simulink model "main_model_fd_v05_energyprotect"  (R2025a)
settings: Solver=ode3  StartTime=0.0  StopTime=1.5  FixedStep=1e-6  RelTol=1e-3
model workspace (MAT data in the model file):
  EP_ENERGY_INITIAL = 176
  EP_PBAT_SIGN = 1
  EP_PLOAD_SIGN = -1
  EP_POWER_ALPHA = 0.951229424501
  EP_POWER_BALANCE_ALPHA = 0.951229424501
  EP_POWER_CONFIRM_TIME = 0.01
  EP_POWER_FILTER_TAU = 0.002
  EP_PSOURCE_SIGN = 1
  EP_P_CHARGE_TRIP = 3000
  EP_P_CHARGE_WARN = 2500
  EP_P_DISCHARGE_TRIP = 3000
  EP_P_DISCHARGE_WARN = 2500
  EP_SOC_CHARGE_RELEASE = 88
  EP_SOC_CHARGE_STOP = 90
  EP_SOC_DISCHARGE_RELEASE = 12
  EP_SOC_DISCHARGE_STOP = 10
  EP_SOC_WARN_HIGH = 85
  EP_SOC_WARN_LOW = 15
  EP_TS = 0.0001
  FD_CBUS = 0.0022
  FD_CBUS_ESR = 0.001
  FD_CURRENT_QUANT_STEP = 1e-06
  FD_DUTY_BIAS = 0
  FD_DUTY_STUCK_ENABLE = 0
  FD_DUTY_STUCK_VALUE = 0.5
  FD_FAULT_END_TIME = 1000000000
  FD_FAULT_ID = 0
  FD_FAULT_TIME = 0.8
  FD_IBAT_BIAS = 0
  FD_IBAT_NOISE_STD = 0
  FD_IBAT_TRIP = 20
  FD_IL_BIAS = 0
  FD_IL_NOISE_STD = 0
  FD_IL_TRIP = 15
  FD_IREF_LEVEL = 10
  FD_IREF_OVERRIDE_ENABLE = 0
  FD_LOAD_STEP_A = 0
  FD_LOAD_STEP_TIME = 0.5
  FD_L_MAIN = 0.015
  FD_MODE_COMMAND = 2
  FD_MODE_OVERRIDE_ENABLE = 0
  FD_PROTECTION_ARM_TIME = 0.15
  FD_PROTECTION_MODE = 2
  FD_RBAT = 0.5
  FD_S1_FAULT_PULSE_WIDTH = 0
  FD_S1_OPEN = 0
  FD_S2_FAULT_PULSE_WIDTH = 0
  FD_S2_OPEN = 0
  FD_SENSOR_TS = 5e-05
  FD_SWITCH_FAULT_PERIOD = 0.0005
  FD_TRIP_DELAY_STEPS = 20000
  FD_TS = 1e-06
  FD_VBAT_BIAS = 0
  FD_VBAT_NOISE_STD = 0
  FD_VBAT_QUANT_STEP = 1e-06
  FD_VBUS_BIAS = 0
  FD_VBUS_HI = 430
  FD_VBUS_LO = 360
  FD_VBUS_NOISE_STD = 0
  FD_VBUS_QUANT_STEP = 1e-06
  I_charge_max = 10
  I_discharge_cmd = 10
  RandomSeed = 240727
  SOCInit = 20
  Var10 = 0
  Var11 = 0
  Var6 = 0
  Var7 = 0
  Var8 = 0
  Var9 = 0
undefined symbols (not defined in the file): DiscIntNeverNeededParam, dspblkCoreblockFVToolHelper, gcbh, Ion, Lithium
libraries: hdlsllib x17, spsSeriesRLCBranchLib x6, spsCurrentMeasurementLib x3, simulink x2, spsIGBTDiodeLib x2, eeGeneralControl x2, slpidlib x2, spsVoltageMeasurementLib x2, spsBatteryLib x1, spsControlledVoltageSourceLib x1, spsControlledCurrentSourceLib x1, spsPWMGeneratorDCDCLib x1
(part 1 of 2)
settings Model: Creator=Limingyu  LastModifiedBy=Administrator
settings DataIOCC: SaveState=on

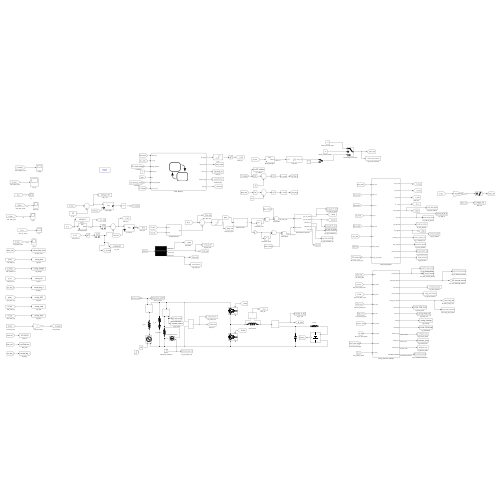
[thumbnail: Simulink's stored preview of the top-level diagram]
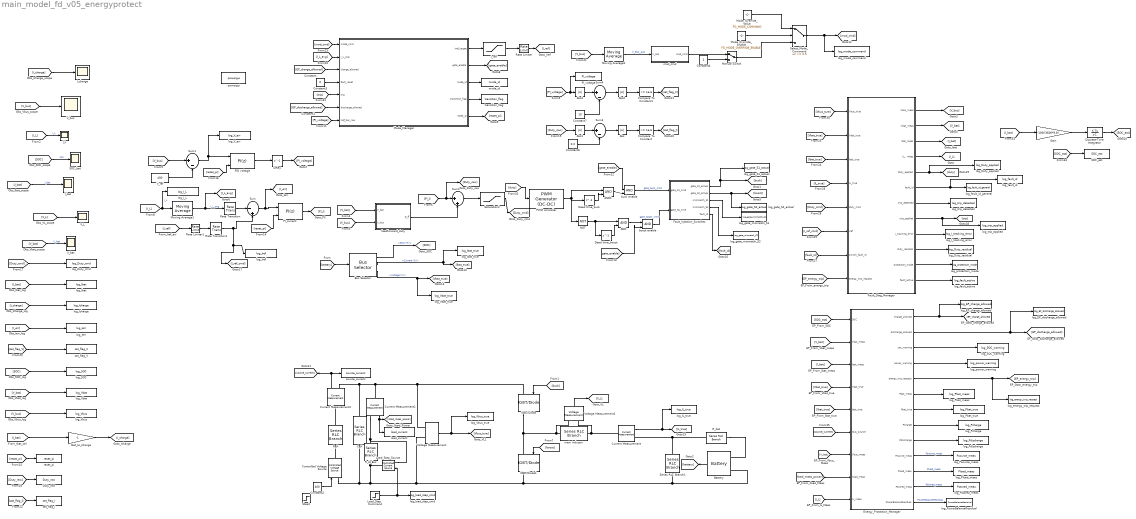
== system main_model_fd_v05_energyprotect ==
  AND : Logic  IconShape=distinctive  AllPortsSameDT=off  OutDataTypeStr=boolean
  AND1 : Logic  IconShape=distinctive  AllPortsSameDT=off  OutDataTypeStr=boolean
  Abs{,1..3} (4 alike) : Abs  SaturateOnIntegerOverflow=off
  Battery : spsBatteryLib/Battery  BatType=Lithium-Ion  NomV=200  NomQ=9.8  SOC=20  Batt_Tr=30  PresetModel=on  MaxQ=9.8  MinV=150  FullV=232.7974  Dis_rate=4.2609  R=0.20408  Normal_OP=8.8626  expZone="[216.0772     0.4814783]"
      link override Model/Discrete/Unit Delay: InitialCondition=Batt.E0 - Batt.K*Batt.Q/(Batt.Q-(1-SOC/100)*Batt.Q*(1/Batt.lambda))*((1-SOC/100)*Batt.Q*(1/Batt.lambda)) + Batt.A*exp(-Batt.B*((1-SOC/100)*Batt.Q*(1/Batt.lambda)))
  Bus Selector : BusSelector  OutputSignals=SOC (%),Current (A),Voltage (V)
  C_H : spsSeriesRLCBranchLib/Series RLC Branch  LConnTagsString=__new0  RConnTagsString=__new0  BranchType=RC  Resistance=FD_CBUS_ESR  Inductance=1e-3  SetiL0=off  InitialCurrent=0  Capacitance=FD_CBUS  Setx0=on  InitialVoltage=400  Measurements=Branch voltage
  Compare To Constant : simulink/Logic and Bit Operations/Compare To Constant  relop=<=  const=1e-6  OutDataTypeStr=boolean
  Compare To Constant1 : simulink/Logic and Bit Operations/Compare To Constant  relop=<=  const=1e-6  OutDataTypeStr=boolean
  Constant2 : Constant  Value=400
  Constant3 : Constant  Value=0  OutDataTypeStr=boolean
  Constant4 : Constant  OutDataTypeStr=double
  Constant6 : Constant  Value=0.2
  Constant7 : Constant  Value=10
  Controlled Voltage Source : spsControlledVoltageSourceLib/Controlled Voltage Source  Initialize=on  Source_Type=DC  Amplitude=400  Phase=0  Frequency=0  Measurements=None
  Current Measurement : spsCurrentMeasurementLib/Current Measurement  PhasorSimulation=off  OutputType=Complex  PSBequivalent=0
  Current Measurement1 : spsCurrentMeasurementLib/Current Measurement  PhasorSimulation=off  OutputType=Complex  PSBequivalent=0
  Current Measurement2 : spsCurrentMeasurementLib/Current Measurement  PhasorSimulation=off  OutputType=Complex  PSBequivalent=0
  Dead time_boost : Delay  DelayLength=1  InputProcessing=Columns as channels (frame based)  SampleTime=2e-6
  Dead time_buck : Delay  DelayLength=1  InputProcessing=Columns as channels (frame based)  SampleTime=2e-6
  Delay : Delay  DelayLength=1  InputProcessing=Columns as channels (frame based)  SampleTime=1e-3
  Discrete-Time Integrator : DiscreteIntegrator  InitialCondition=SOCInit  SampleTime=EP_TS  LimitOutput=on  UpperSaturationLimit=100  LowerSaturationLimit=0  ICPrevOutput=DiscIntNeverNeededParam  ICPrevScaledInput=DiscIntNeverNeededParam
  Duty_raw : ToWorkspace  VariableName=Duty_raw  SaveFormat=Timeseries  SampleTime=-1
  Energy_Protection_Manager : Subsystem
  Fault_Diag_Manager : Subsystem
  Fault_Injection_Switches : Subsystem
  Gain : Gain  Gain=-100/(3600*9.8)
  IGBT/Diode : spsIGBTDiodeLib/IGBT//Diode  Ron=1e-3  Rs=1e5  Cs=inf  Measurements=on
  IGBT/Diode1 : spsIGBTDiodeLib/IGBT//Diode  Ron=1e-3  Rs=1e5  Cs=inf  Measurements=on
  I_L : Scope
      settings: ActiveDisplayYMinimum=-1  ActiveDisplayYMaximum=1
  I_bat : Scope
      settings: ActiveDisplayYMinimum=9.9262651650151241  ActiveDisplayYMaximum=26.223015826126126  DataLoggingVariableName=scope_V_bat1
  I_charge : Scope
      settings: ActiveDisplayYMinimum=-1435.850063928573  ActiveDisplayYMaximum=6954.7870735806873  DataLoggingVariableName=scope_I_L
  I_ref' : Saturate  UpperLimit=I_charge_max  LowerLimit=-I_discharge_cmd
  Ibat_to_Icharge : Gain  Gain=-1
  Load_Step_Command : Step  Time=FD_LOAD_STEP_TIME  After=FD_LOAD_STEP_A  SampleTime=FD_TS
  Load_Step_Source : spsControlledCurrentSourceLib/Controlled Current Source  Initialize=on  Source_Type=AC  Amplitude=0  Phase=0  Frequency=0  Measurements=None
  Manual Switch : ManualSwitch
  Mode_Manager : Stateflow chart  TreatAsAtomicUnit=on
  Mode_Override_Enable : Constant  Value=FD_MODE_OVERRIDE_ENABLE
  Mode_Override_Value : Constant  Value=FD_MODE_COMMAND
  Moving Average1 : eeGeneralControl/Moving Average  VariantControl=Variant1  LabelModeActiveChoice=Discrete  f=20e3  x0=0  BufferSize=8192  Ts=1e-6
      settings: LibrarySourceBlock=ee_sl_lib/General Control/Moving Average
  Moving Average2 : eeGeneralControl/Moving Average  VariantControl=Variant1  LabelModeActiveChoice=Discrete  f=20e3  x0=0  BufferSize=8192  Ts=1e-6
      settings: LibrarySourceBlock=ee_sl_lib/General Control/Moving Average
  NOT : Logic  Operator=NOT  IconShape=distinctive  AllPortsSameDT=off  OutDataTypeStr=boolean
  PID voltage : slpidlib/PID Controller  Controller=PI  Form=Parallel  TimeDomain=Discrete-time  UseExternalTs=off  SampleTime=1e-3  IntegratorMethod=Forward Euler  FilterMethod=Forward Euler  ControllerParametersSource=internal  P=2.6  I=50  UseKiTs=off  D=0  UseExternalDerivativeSource=off  N=100  UseFilter=on  TunerSelectOption=Transfer Function Based (PID Tuner App)  InitialConditionSource=internal  InitialConditionForIntegrator=0  InitialConditionForFilter=0  DifferentiatorICPrevScaledInput=0  ExternalReset=rising  TrackingMode=off  Kt=1  LimitOutput=on  SatLimitsSource=internal  UpperSaturationLimit=10  LowerSaturationLimit=-10  LinearizeAsGain=on  AntiWindupMode=back-calculation  Kb=20  LimitIntegrator=off  UpperIntegratorSaturationLimit=inf  LowerIntegratorSaturationLimit=-inf  POutMin=[]  POutMax=[]  IOutMin=[]  IOutMax=[]  DOutMin=[]  DOutMax=[]  NOutMin=[]  NOutMax=[]  SumOutMin=[]  SumOutMax=[]  SaturationOutMin=[]  SaturationOutMax=[]  PParamMin=[]  PParamMax=[]  IParamMin=[]  IParamMax=[]  DParamMin=[]  DParamMax=[]  NParamMin=[]  NParamMax=[]  KbParamMin=[]  KbParamMax=[]  KtParamMin=[]  KtParamMax=[]  KbOutMin=[]  KbOutMax=[]  KtOutMin=[]  KtOutMax=[]  IntegratorOutMin=[]  IntegratorOutMax=[]  FilterOutMin=[]  FilterOutMax=[]  SumI1OutMin=[]  SumI1OutMax=[]  SumI2OutMin=[]  SumI2OutMax=[]  SumI3OutMin=[]  SumI3OutMax=[]  SumI4OutMin=[]  SumI4OutMax=[]  SumDOutMin=[]  SumDOutMax=[]  DifferentiatorOutMin=[]  DifferentiatorOutMax=[]  FilterDiffOutCoefMin=[]  FilterDiffOutCoefMax=[]  ReciprocalOutMin=[]  ReciprocalOutMax=[]  SumDenOutMin=[]  SumDenOutMax=[]  SumNumOutMin=[]  SumNumOutMax=[]  DivideOutMin=[]  DivideOutMax=[]  UdiffTsProdOutMin=[]  UdiffTsProdOutMax=[]  NTsProdOutMin=[]  NTsProdOutMax=[]  UintegralTsProdOutMin=[]  UintegralTsProdOutMax=[]  UngainTsProdOutMin=[]  UngainTsProdOutMax=[]  ClampingZeroOutDataTypeStr=Inherit: Inherit via back propagation  ClampingZeroOutMin=[]  ClampingZeroOutMax=[]  FilterDenConstantOutDataTypeStr=Inherit: Inherit via back propagation  FilterDenConstantOutMin=[]  FilterDenConstantOutMax=[]  PCopyOutDataTypeStr=Inherit: Inherit via back propagation  PCopyOutMin=[]  PCopyOutMax=[]  NCopyOutDataTypeStr=Inherit: Inherit via back propagation  NCopyOutMin=[]  NCopyOutMax=[]  IntegratorContinuousStateAttributes=''  IntegratorStateMustResolveToSignalObject=off  IntegratorRTWStateStorageClass=Auto  FilterContinuousStateAttributes=''  FilterStateMustResolveToSignalObject=off  FilterRTWStateStorageClass=Auto  ParallelPVariant=InternalParameters  IdealPVariant=Disabled  IVariant=InternalParameters  DVariant=Disabled  IntegratorVariant=Discrete  SatVariant=Enabled  AWVariant=BackCalculation  PCopyVariant=Disabled  TRVariant=Disabled  FdbkBlocksVariant=Forward  IdealPFdbkVariant=Disabled  SatFdbkVariant=Disabled  DerivativeFilterVariant=Disabled  NVariant=Disabled  NCopyVariant=Disabled_SignalSpec  FilterICVariant=Disabled  IntegratorICVariant=InternalICs  ExternalResetVariant=ExternalReset  TRSumVariant=Passthrough  SumFdbkVariant=Disabled  SumVariant=Sum_PI  TsampFilterVariant=InternalTs  TsampNgainVariant=Passthrough  TsampIntegralVariant=Disabled_SignalSpec  ExternalSaturationOutDataTypeStr=Inherit: Same as second input  DerivativeSourceVariant=Disabled  PreIntVariant=InternalPreInt
  PI_current : slpidlib/PID Controller  Controller=PI  Form=Parallel  TimeDomain=Discrete-time  UseExternalTs=off  SampleTime=50e-6  IntegratorMethod=Forward Euler  FilterMethod=Forward Euler  ControllerParametersSource=internal  P=0.236  I=50  UseKiTs=off  D=0  UseExternalDerivativeSource=off  N=100  UseFilter=on  TunerSelectOption=Transfer Function Based (PID Tuner App)  InitialConditionSource=internal  InitialConditionForIntegrator=0  InitialConditionForFilter=0  DifferentiatorICPrevScaledInput=0  ExternalReset=rising  TrackingMode=off  Kt=1  LimitOutput=on  SatLimitsSource=internal  UpperSaturationLimit=0.2  LowerSaturationLimit=-0.2  LinearizeAsGain=on  AntiWindupMode=back-calculation  Kb=100  LimitIntegrator=off  UpperIntegratorSaturationLimit=inf  LowerIntegratorSaturationLimit=-inf  POutMin=[]  POutMax=[]  IOutMin=[]  IOutMax=[]  DOutMin=[]  DOutMax=[]  NOutMin=[]  NOutMax=[]  SumOutMin=[]  SumOutMax=[]  SaturationOutMin=[]  SaturationOutMax=[]  PParamMin=[]  PParamMax=[]  IParamMin=[]  IParamMax=[]  DParamMin=[]  DParamMax=[]  NParamMin=[]  NParamMax=[]  KbParamMin=[]  KbParamMax=[]  KtParamMin=[]  KtParamMax=[]  KbOutMin=[]  KbOutMax=[]  KtOutMin=[]  KtOutMax=[]  IntegratorOutMin=[]  IntegratorOutMax=[]  FilterOutMin=[]  FilterOutMax=[]  SumI1OutMin=[]  SumI1OutMax=[]  SumI2OutMin=[]  SumI2OutMax=[]  SumI3OutMin=[]  SumI3OutMax=[]  SumI4OutMin=[]  SumI4OutMax=[]  SumDOutMin=[]  SumDOutMax=[]  DifferentiatorOutMin=[]  DifferentiatorOutMax=[]  FilterDiffOutCoefMin=[]  FilterDiffOutCoefMax=[]  ReciprocalOutMin=[]  ReciprocalOutMax=[]  SumDenOutMin=[]  SumDenOutMax=[]  SumNumOutMin=[]  SumNumOutMax=[]  DivideOutMin=[]  DivideOutMax=[]  UdiffTsProdOutMin=[]  UdiffTsProdOutMax=[]  NTsProdOutMin=[]  NTsProdOutMax=[]  UintegralTsProdOutMin=[]  UintegralTsProdOutMax=[]  UngainTsProdOutMin=[]  UngainTsProdOutMax=[]  ClampingZeroOutDataTypeStr=Inherit: Inherit via back propagation  ClampingZeroOutMin=[]  ClampingZeroOutMax=[]  FilterDenConstantOutDataTypeStr=Inherit: Inherit via back propagation  FilterDenConstantOutMin=[]  FilterDenConstantOutMax=[]  PCopyOutDataTypeStr=Inherit: Inherit via back propagation  PCopyOutMin=[]  PCopyOutMax=[]  NCopyOutDataTypeStr=Inherit: Inherit via back propagation  NCopyOutMin=[]  NCopyOutMax=[]  IntegratorContinuousStateAttributes=''  IntegratorStateIdentifier=PIiIntegral  IntegratorStateMustResolveToSignalObject=off  IntegratorRTWStateStorageClass=Auto  FilterContinuousStateAttributes=''  FilterStateMustResolveToSignalObject=off  FilterRTWStateStorageClass=Auto  ParallelPVariant=InternalParameters  IdealPVariant=Disabled  IVariant=InternalParameters  DVariant=Disabled  IntegratorVariant=Discrete  SatVariant=Enabled  AWVariant=BackCalculation  PCopyVariant=Disabled  TRVariant=Disabled  FdbkBlocksVariant=Forward  IdealPFdbkVariant=Disabled  SatFdbkVariant=Disabled  DerivativeFilterVariant=Disabled  NVariant=Disabled  NCopyVariant=Disabled_SignalSpec  FilterICVariant=Disabled  IntegratorICVariant=InternalICs  ExternalResetVariant=ExternalReset  TRSumVariant=Passthrough  SumFdbkVariant=Disabled  SumVariant=Sum_PI  TsampFilterVariant=InternalTs  TsampNgainVariant=Passthrough  TsampIntegralVariant=Disabled_SignalSpec  ExternalSaturationOutDataTypeStr=Inherit: Same as second input  DerivativeSourceVariant=Disabled  PreIntVariant=InternalPreInt
  PI_voltage : ToWorkspace  VariableName=PI_voltage  SaveFormat=Timeseries  SampleTime=-1
  PWM controller : spsPWMGeneratorDCDCLib/PWM Generator (DC-DC)  Fsw=20e3  Ts=1e-6
  R_H : spsSeriesRLCBranchLib/Series RLC Branch  LConnTagsString=__new0  RConnTagsString=__new0  BranchType=R  Resistance=2  Inductance=1e-3  SetiL0=off  InitialCurrent=0  Capacitance=1e-6  Setx0=off  InitialVoltage=0  Measurements=Branch voltage and current
  R_H_Bus : spsSeriesRLCBranchLib/Series RLC Branch  LConnTagsString=__new0  RConnTagsString=__new0  BranchType=R  Resistance=200  Inductance=1e-3  SetiL0=off  InitialCurrent=0  Capacitance=1e-6  Setx0=off  InitialVoltage=0  Measurements=None
  R_bat : spsSeriesRLCBranchLib/Series RLC Branch  LConnTagsString=__new0  RConnTagsString=__new0  BranchType=R  Resistance=FD_RBAT  Inductance=1e-3  SetiL0=off  InitialCurrent=0  Capacitance=1e-6  Setx0=off  InitialVoltage=0  Measurements=None
  Rate Limiter : RateLimiter  RisingSlewLimit=200  FallingSlewLimit=-200  SampleTimeMode=inherited
  Rate Limiter1 : RateLimiter  RisingSlewLimit=200  FallingSlewLimit=-200  SampleTimeMode=inherited
  Rate Transition : RateTransition
  Rate Transition1 : RateTransition  Deterministic=off  OutPortSampleTime=50E-6
  SOC_bat : Scope
      settings: ActiveDisplayYMinimum=9.9262651650151241  ActiveDisplayYMaximum=26.223015826126126  DataLoggingVariableName=scope_V_bat2
  SOC_est : ToWorkspace  VariableName=SOC_est  SaveFormat=Timeseries  SampleTime=-1
  Saturation2 : Saturate  UpperLimit=1  LowerLimit=0
  Select_Mode_Command : Switch  Threshold=0.5
  Series RLC Branch1 : spsSeriesRLCBranchLib/Series RLC Branch  LConnTagsString=__new0  RConnTagsString=__new0  BranchType=C  Resistance=1  Inductance=1e-3  SetiL0=off  InitialCurrent=0  Capacitance=1e-3  Setx0=on  InitialVoltage=200  Measurements=None
  Step2 : Step  Time=0.1  Before=396  After=414  SampleTime=0
  Sum : Sum  Inputs=|-+
  Sum1 : Sum  Inputs=|+-
  Sum2 : Sum  Inputs=|++
  Sum3 : Sum  Inputs=|+-
  Sum4 : Sum  Inputs=|+-
  V_L : Scope
      settings: ActiveDisplayYMinimum=1.7818295198342415  ActiveDisplayYMaximum=30.840341432126138  DataLoggingVariableName=scope_V_L
  V_bat : Scope
      settings: ActiveDisplayYMinimum=9.9262651650151241  ActiveDisplayYMaximum=26.223015826126126  DataLoggingVariableName=scope_V_bat
  V_bus : Scope
      settings: ActiveDisplayYMinimum=35.013513154974092  ActiveDisplayYMaximum=46.766305604047623  DataLoggingVariableName=scope_V_bus
  V_ref : Constant  Value=400
  Voltage Measurement : spsVoltageMeasurementLib/Voltage Measurement  PhasorSimulation=off  OutputType=Complex  PSBequivalent=0
  Voltage Measurement2 : spsVoltageMeasurementLib/Voltage Measurement  PhasorSimulation=off  OutputType=Complex  PSBequivalent=0
  boost enable : Logic  IconShape=distinctive  AllPortsSameDT=off  OutDataTypeStr=boolean
  buck enable : Logic  IconShape=distinctive  AllPortsSameDT=off  OutDataTypeStr=boolean
  feedforward_duty : Subsystem
  load_current : ToWorkspace  VariableName=load_current  SaveFormat=Timeseries  SampleTime=-1
  log_Duty_applied : ToWorkspace  VariableName=log_Duty_applied  SaveFormat=Timeseries  SampleTime=-1
      settings: Decimation=20
  log_Duty_cmd : ToWorkspace  VariableName=log_Duty_cmd  SaveFormat=Timeseries  SampleTime=-1
  log_Duty_residual : ToWorkspace  VariableName=log_Duty_residual  SaveFormat=Timeseries  SampleTime=-1
      settings: Decimation=20
  log_EP_charge_allowed : ToWorkspace  VariableName=log_EP_charge_allowed  SaveFormat=Timeseries
  log_EP_discharge_allowed : ToWorkspace  VariableName=log_EP_discharge_allowed  SaveFormat=Timeseries
  log_IL_true : ToWorkspace  VariableName=log_IL_true  SaveFormat=Timeseries  SampleTime=-1
      settings: Decimation=20
  log_I_L : ToWorkspace  VariableName=log_I_L  SaveFormat=Timeseries  SampleTime=-1
      settings: Decimation=20
  log_I_tracking_error : ToWorkspace  VariableName=log_I_tracking_error  SaveFormat=Timeseries  SampleTime=-1
      settings: Decimation=20
  log_Ibat : ToWorkspace  VariableName=log_Ibat  SaveFormat=Timeseries  SampleTime=-1
      settings: Decimation=20
  log_Ibat_true : ToWorkspace  VariableName=log_Ibat_true  SaveFormat=Timeseries  SampleTime=-1
      settings: Decimation=20
  log_Icharge : ToWorkspace  VariableName=log_Icharge  SaveFormat=Timeseries  SampleTime=-1
  log_Ierr : ToWorkspace  VariableName=log_Ierr  SaveFormat=Timeseries  SampleTime=-1
  log_Iref : ToWorkspace  VariableName=log_Iref  SaveFormat=Timeseries  SampleTime=-1
  log_Pbat_meas : ToWorkspace  VariableName=log_Pbat_meas  SaveFormat=Timeseries
  log_Pbat_true : ToWorkspace  VariableName=log_Pbat_true  SaveFormat=Timeseries
  log_Pcharge : ToWorkspace  VariableName=log_Pcharge  SaveFormat=Timeseries
  log_Pdischarge : ToWorkspace  VariableName=log_Pdischarge  SaveFormat=Timeseries
  log_Pload_meas : ToWorkspace  VariableName=Pload_meas  SaveFormat=Timeseries  SampleTime=-1
  log_PowerBalanceResidual : ToWorkspace  VariableName=PowerBalanceResidual  SaveFormat=Timeseries  SampleTime=-1
  log_Psource_meas : ToWorkspace  VariableName=Psource_meas  SaveFormat=Timeseries  SampleTime=-1
  log_Pstored_meas : ToWorkspace  VariableName=Pstored_meas  SaveFormat=Timeseries  SampleTime=-1
  log_SOC : ToWorkspace  VariableName=log_SOC  SaveFormat=Timeseries
      settings: Decimation=1000
  log_SOC_warning : ToWorkspace  VariableName=log_SOC_warning  SaveFormat=Timeseries
  log_V_err : ToWorkspace  VariableName=log_V_err  SaveFormat=Timeseries  SampleTime=-1
  log_Vbat : ToWorkspace  VariableName=log_Vbat  SaveFormat=Timeseries
      settings: Decimation=20
  log_Vbat_true : ToWorkspace  VariableName=log_Vbat_true  SaveFormat=Timeseries  SampleTime=-1
      settings: Decimation=20
  log_Vbus : ToWorkspace  VariableName=log_Vbus  SaveFormat=Timeseries
      settings: Decimation=20
  log_Vbus_true : ToWorkspace  VariableName=log_Vbus_true  SaveFormat=Timeseries  SampleTime=-1
      settings: Decimation=20
  log_energy_trip_request : ToWorkspace  VariableName=log_energy_trip_request  SaveFormat=Timeseries
  log_fault_active : ToWorkspace  VariableName=log_fault_active  SaveFormat=Timeseries  SampleTime=-1
      settings: Decimation=20
  log_fault_id : ToWorkspace  VariableName=log_fault_id  SaveFormat=Timeseries
      settings: Decimation=20
  log_fault_id_general : ToWorkspace  VariableName=log_fault_id_general  SaveFormat=Timeseries  SampleTime=-1
      settings: Decimation=20
  log_gate_S1_actual : ToWorkspace  VariableName=log_gate_S1_actual  SaveFormat=Timeseries
      settings: Decimation=20
  log_gate_S2_actual : ToWorkspace  VariableName=log_gate_S2_actual  SaveFormat=Timeseries
      settings: Decimation=20
  log_gate_mismatch_S1 : ToWorkspace  VariableName=log_gate_mismatch_S1  SaveFormat=Timeseries
      settings: Decimation=20
  log_gate_mismatch_S2 : ToWorkspace  VariableName=log_gate_mismatch_S2  SaveFormat=Timeseries
      settings: Decimation=20
  log_load_step_cmd : ToWorkspace  VariableName=log_load_step_cmd  SaveFormat=Timeseries  SampleTime=-1
      settings: Decimation=20
  log_mode_command : ToWorkspace  VariableName=log_mode_command  SaveFormat=Timeseries  SampleTime=-1
  log_power_warning : ToWorkspace  VariableName=log_power_warning  SaveFormat=Timeseries
  log_protection_mode : ToWorkspace  VariableName=log_protection_mode  SaveFormat=Timeseries  SampleTime=-1
      settings: Decimation=20
  log_trip_applied : ToWorkspace  VariableName=log_trip_applied  SaveFormat=Timeseries  SampleTime=-1
      settings: Decimation=20
  log_trip_detected : ToWorkspace  VariableName=log_trip_detected  SaveFormat=Timeseries  SampleTime=-1
      settings: Decimation=20
  main inductor : spsSeriesRLCBranchLib/Series RLC Branch  LConnTagsString=__new0  RConnTagsString=__new0  BranchType=L  Resistance=1  Inductance=15e-3  SetiL0=off  InitialCurrent=0  Capacitance=1e-6  Setx0=off  InitialVoltage=0  Measurements=None
  mod_cmd : Stateflow chart  TreatAsAtomicUnit=on
  mode_id : ToWorkspace  VariableName=mode_id  SaveFormat=Timeseries  SampleTime=-1
  powergui : sps_lib/powergui  Priority=1  SimulationMode=Discrete  SampleTime=1e-6  frequency=60  Iterations=50  frequencyindice=0  Pbase=100e6  ErrMax=1e-4  UnitsV=kV  UnitsW=MW  buscounter=0  FunctionMessages=off  echomessages=off  EnableUseOfTLC=off  CurrentSourceSwitches=off  DisableSnubberDevices=off  DisableRonSwitches=off  DisableVfSwitches=off  DisplayEquations=off  AutomaticDiscreteSolvers=off  SolverType=Tustin/Backward Euler (TBE)  Interpol=off  ExternalGateDelay=off  methode=off  Ts=100  x0status=blocks  SPID=on  SwTol=0  HookPort=off  NonlinearTolerance=1e-4  nMaxIteration=100  ContinueOnMaxIteration=off  RestoreLinks=warning  ResistiveCurrentMeasurement=off  Frange=[0:2:500]  Ylog=off  Xlog=on  ShowGrid=off  save=off  variable=ZData  structure=0  ZoomFFT=off  StartTime=0.0  cycles=1  DisplayStyle=1  fundamental=60  FreqAxis=off  MaxFrequency=1000  frequencyindicesteady=1  RmsSteady=1  display=off
  reset_pi : ToWorkspace  VariableName=reset_pi  SaveFormat=Timeseries  SampleTime=-1
  sat_flag_I : ToWorkspace  VariableName=sat_flag_I  SaveFormat=Timeseries  SampleTime=-1
  sat_flag_V : ToWorkspace  VariableName=sat_flag_V  SaveFormat=Timeseries  SampleTime=-1
  source_current : ToWorkspace  VariableName=source_current  SaveFormat=Timeseries  SampleTime=-1
  transition_flag : ToWorkspace  VariableName=transition_flag  SaveFormat=Timeseries  SampleTime=-1
  wires:
  Sum1/1 -> log_V_err/1, PID voltage/1
  V_ref/1 -> Sum1/2
  [V_bat] -> feedforward_duty/1(V_bat)
  [V_bus] -> feedforward_duty/2(V_bus)
  PWM controller/1 -> AND1/1, Dead time_buck/1, NOT/1
  [I_bat] -> Ibat_to_Icharge/1
  [I_charge] -> I_charge/1
  [V_bus] -> V_bus/1
  [V_bat] -> V_bat/1  "V_bat"
  [I_bat] -> I_bat/1  "I_bat"
  [V_L] -> V_L/1
  [SOC] -> log_SOC/1
  [I_bat] -> log_Ibat/1
  [V_bat] -> log_Vbat/1
  [I_charge] -> log_Icharge/1
  [V_bus] -> log_Vbus/1
  [Duty_cmd] -> log_Duty_cmd/1
  [I_err] -> log_Ierr/1
  Saturation2/1 -> [Duty_cmd]
  Bus Selector/1 -> [SOC]  "<SOC (%)>"
  Voltage Measurement2/1 -> [V_L]
  Battery/1 -> [battery]
  [battery] -> Bus Selector/1
  Ibat_to_Icharge/1 -> [I_charge]
  [SOC] -> SOC_bat/1  "soc"
  [I_L] -> I_L/1  "I_L"
  Sum/1 -> [I_err], PI_current/1
  PI_current/1 -> [PI_I]
  [PI_I] -> [Duty_raw], Sum2/1
  feedforward_duty/1(D_ff) -> Sum2/2
  Sum2/1 -> Saturation2/1
  NOT/1 -> Dead time_boost/1, AND/1
  Dead time_boost/1 -> AND/2
  Dead time_buck/1 -> AND1/2
  [buck] -> IGBT/Diode/1
  [boost] -> IGBT/Diode1/1
  [I_L] -> Moving Average1/1, log_I_L/1  "I_L"
  AND1/1 -> buck enable/2
  AND/1 -> boost enable/1
  Moving Average1/1 -> Rate Transition/1, [I_L_avg]  "I_L_avg"
  Rate Transition/1 -> Sum/1
  Constant3/1 -> Mode_Manager/4(fault_reset)
  [I_L_avg] -> Mode_Manager/2(I_L_avg)
  Mode_Manager/2(gate_enable) -> [gate_enable]
  [gate_enable] -> buck enable/1
  [gate_enable] -> boost enable/2
  Mode_Manager/3(mode_id) -> mode_id/1
  Mode_Manager/4(transition_flag) -> transition_flag/1
  Mode_Manager/5(reset_pi) -> [reset_pi]
  [reset_pi] -> PI_current/2
  [reset_pi] -> reset_pi/1
  [V_bus] -> Sum1/1
  [reset_pi] -> PID voltage/2
  PID voltage/1 -> Delay/1
  [Duty_raw] -> Duty_raw/1
  [Duty_raw] -> Abs1/1
  Sum3/1 -> Abs/1
  Abs/1 -> Compare To Constant/1
  Compare To Constant/1 -> [sat_flag_I]
  [sat_flag_I] -> sat_flag_I/1
  [PI_voltage] -> Mode_Manager/7(Iref_bus_raw)
  I_ref'/1 -> Rate Limiter/1
  Constant6/1 -> Sum3/2
  Abs1/1 -> Sum3/1
  Rate Transition1/1 -> [I_ref_cmd], log_Iref/1, Sum/2
  Mode_Manager/1(Iref_target) -> I_ref'/1
  Rate Limiter/1 -> [I_ref]
  Delay/1 -> [PI_voltage]
  Rate Limiter1/1 -> Rate Transition1/1
  [I_ref] -> Rate Limiter1/1
  Current Measurement1/1 -> load_current/1, [Iload_meas_power]
  buck enable/1 -> Fault_Injection_Switches/1(gate_S1_cmd)  "gate_buck_cmd"
  boost enable/1 -> Fault_Injection_Switches/2(gate_S2_cmd)  "gate_boost_cmd"
  Fault_Injection_Switches/1(gate_S1_actual) -> log_gate_S1_actual/1, [buck]
  Fault_Injection_Switches/2(gate_S2_actual) -> [boost], log_gate_S2_actual/1
  Fault_Injection_Switches/3(mismatch_S1) -> log_gate_mismatch_S1/1
  Fault_Injection_Switches/4(mismatch_S2) -> log_gate_mismatch_S2/1
  Abs3/1 -> Sum4/1
  Compare To Constant1/1 -> [sat_flag_V]
  [PI_voltage] -> PI_voltage/1, Abs3/1
  Abs2/1 -> Compare To Constant1/1
  Constant7/1 -> Sum4/2
  Sum4/1 -> Abs2/1
  [sat_flag_V] -> sat_flag_V/1
  [V_bus] -> Moving Average2/1
  Constant4/1 -> Manual Switch/2
  mod_cmd/1(mod_cmd) -> Manual Switch/1
  Moving Average2/1 -> mod_cmd/1(V_bus)  "V_Bus_avg"
  Voltage Measurement/1 -> [Vbus_ture], log_Vbus_true/1
  Fault_Diag_Manager/1(Vbus_meas) -> [V_bus]
  Bus Selector/3 -> [Vbat_true], log_Vbat_true/1  "<Voltage (V)>"
  Fault_Diag_Manager/2(Vbat_meas) -> [V_bat]
  Bus Selector/2 -> [Ibat_true], log_Ibat_true/1  "<Current (A)>"
  Fault_Diag_Manager/3(Ibat_meas) -> [I_bat]
  Current Measurement/1 -> [IL_true], log_IL_true/1
  Fault_Diag_Manager/4(IL_  meas) -> [I_L]
  Fault_Diag_Manager/5(Duty_applied) -> log_Duty_applied/1, [duty]
  Fault_Diag_Manager/6(fault_id) -> log_fault_id/1, log_fault_id_general/1
  Fault_Diag_Manager/7(trip_detected) -> log_trip_detected/1
  Fault_Diag_Manager/9(I_tracking_error) -> log_I_tracking_error/1
  Fault_Diag_Manager/10(Duty_residual) -> log_Duty_residual/1
  Fault_Diag_Manager/11(protection_mode) -> log_protection_mode/1
  Fault_Diag_Manager/12(fault_active) -> log_fault_active/1
  Load_Step_Command/1 -> log_load_step_cmd/1, Load_Step_Source/1
  Mode_Override_Value/1 -> Select_Mode_Command/1
  Mode_Override_Enable/1 -> Select_Mode_Command/2
  Manual Switch/1 -> Select_Mode_Command/3
  Select_Mode_Command/1 -> [mod_cmd], log_mode_command/1
  [Ibat_true] -> Fault_Diag_Manager/3(Ibat_true)
  [Vbat_true] -> Fault_Diag_Manager/2(Vbat_true)
  [IL_true] -> Fault_Diag_Manager/4(IL_true)
  Fault_Injection_Switches/5(fault_id) -> [fault_id]
  [fault_id] -> Fault_Diag_Manager/7(switch_fault_id)
  [Duty_cmd] -> Fault_Diag_Manager/5(Duty_cmd)
  [I_ref_cmd] -> Fault_Diag_Manager/6(Iref)
  [Vbus_ture] -> Fault_Diag_Manager/1(Vbus_true)
  Fault_Diag_Manager/8(trip_applied) -> log_trip_applied/1, [trip]
  [trip] -> Mode_Manager/5(trip)
  [mod_cmd] -> Mode_Manager/1(mode_cmd)
  [duty] -> PWM controller/1
  [SOC_est] -> Energy_Protection_Manager/1(SOC)
  [V_bat] -> Energy_Protection_Manager/2(Vbat_meas)
  [I_bat] -> Energy_Protection_Manager/3(Ibat_meas)
  [Vbat_true] -> Energy_Protection_Manager/4(Vbat_true)
  [Ibat_true] -> Energy_Protection_Manager/5(Ibat_true)
  Energy_Protection_Manager/1(charge_allowed) -> [EP_charge_allowed], log_EP_charge_allowed/1
  Energy_Protection_Manager/2(discharge_allowed) -> [EP_discharge_allowed], log_EP_discharge_allowed/1
  Energy_Protection_Manager/3(soc_warning) -> log_SOC_warning/1
  Energy_Protection_Manager/4(power_warning) -> log_power_warning/1
  Energy_Protection_Manager/5(energy_trip_request) -> log_energy_trip_request/1, [EP_energy_trip]
  Energy_Protection_Manager/6(Pbat_meas) -> log_Pbat_meas/1
  Energy_Protection_Manager/7(Pbat_true) -> log_Pbat_true/1
  Energy_Protection_Manager/8(Pcharge) -> log_Pcharge/1
  Energy_Protection_Manager/9(Pdischarge) -> log_Pdischarge/1
  [EP_charge_allowed] -> Mode_Manager/3(charge_allowed)
  [EP_discharge_allowed] -> Mode_Manager/6(discharge_allowed)
  [EP_energy_trip] -> Fault_Diag_Manager/8(energy_trip_request)
  [I_bat] -> Gain/1
  Gain/1 -> Discrete-Time Integrator/1
  Discrete-Time Integrator/1 -> [SOC_est]
  [SOC_est] -> SOC_est/1
  Current Measurement2/1 -> source_current/1, [source_current]
  [source_current] -> Energy_Protection_Manager/6(Ibus_source)
  [V_bus] -> Energy_Protection_Manager/7(Vbus_meas)
  [Iload_meas_power] -> Energy_Protection_Manager/8(Iload_meas)
  [I_L] -> Energy_Protection_Manager/9(IL_meas)
  Energy_Protection_Manager/10(Psource_meas) -> log_Psource_meas/1  "Psource_meas"
  Energy_Protection_Manager/11(Pload_meas) -> log_Pload_meas/1  "Pload_meas"
  Energy_Protection_Manager/12(Pstored_meas) -> log_Pstored_meas/1  "Pstored_meas"
  Energy_Protection_Manager/13(PowerBalanceResidual) -> log_PowerBalanceResidual/1  "PowerBalanceResidual"
  Constant2/1 -> Controlled Voltage Source/1
  connections:
  Voltage Measurement/LConn1 -- IGBT/Diode/LConn1 -- Current Measurement1/LConn1 -- C_H/LConn1 -- Current Measurement2/RConn1
  C_H/RConn1 -- R_H_Bus/RConn1 -- Load_Step_Source/RConn1 -- Voltage Measurement/LConn2 -- IGBT/Diode1/RConn1 -- Series RLC Branch1/RConn1 -- Battery/LConn2 -- Controlled Voltage Source/LConn1
  IGBT/Diode/RConn1 -- Voltage Measurement2/LConn1 -- main inductor/LConn1 -- IGBT/Diode1/LConn1
  Voltage Measurement2/LConn2 -- Current Measurement/LConn1 -- main inductor/RConn1
  Series RLC Branch1/LConn1 -- Current Measurement/RConn1 -- R_bat/RConn1
  R_bat/LConn1 -- Battery/LConn1
  Current Measurement1/RConn1 -- Load_Step_Source/LConn1 -- R_H_Bus/LConn1
  Controlled Voltage Source/RConn1 -- R_H/RConn1
  R_H/LConn1 -- Current Measurement2/LConn1

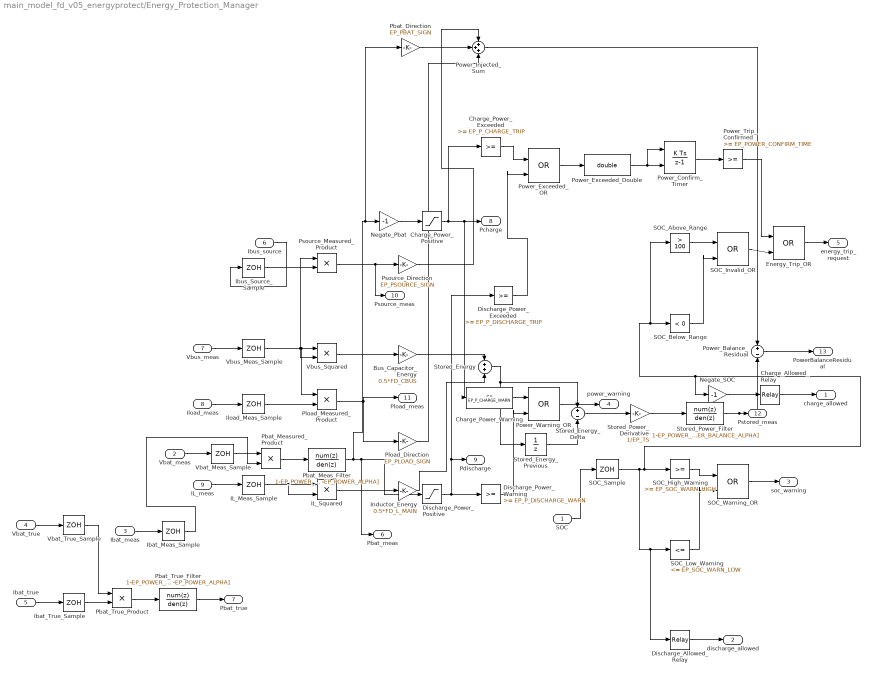
== system main_model_fd_v05_energyprotect/Energy_Protection_Manager ==
  SOC : Inport
  Vbat_meas : Inport  Port=2
  Ibat_meas : Inport  Port=3
  Vbat_true : Inport  Port=4
  Ibat_true : Inport  Port=5
  Ibus_source : Inport  Port=6
  Vbus_meas : Inport  Port=7
  Iload_meas : Inport  Port=8
  IL_meas : Inport  Port=9
  Bus_Capacitor_Energy : Gain  Gain=0.5*FD_CBUS
  Charge_Allowed_Relay : Relay  OnSwitchValue=-EP_SOC_CHARGE_RELEASE  OffSwitchValue=-EP_SOC_CHARGE_STOP  OutDataTypeStr=boolean
  Charge_Power_Exceeded : hdlsllib/Logic and Bit Operations/Compare To Constant  relop=>=  const=EP_P_CHARGE_TRIP  OutDataTypeStr=boolean
  Charge_Power_Positive : Saturate  UpperLimit=inf  LowerLimit=0
  Charge_Power_Warning : hdlsllib/Logic and Bit Operations/Compare To Constant  relop=>=  const=EP_P_CHARGE_WARN  OutDataTypeStr=boolean
  Discharge_Allowed_Relay : Relay  OnSwitchValue=EP_SOC_DISCHARGE_RELEASE  OffSwitchValue=EP_SOC_DISCHARGE_STOP  OutDataTypeStr=boolean
  Discharge_Power_Exceeded : hdlsllib/Logic and Bit Operations/Compare To Constant  relop=>=  const=EP_P_DISCHARGE_TRIP  OutDataTypeStr=boolean
  Discharge_Power_Positive : Saturate  UpperLimit=inf  LowerLimit=0
  Discharge_Power_Warning : hdlsllib/Logic and Bit Operations/Compare To Constant  relop=>=  const=EP_P_DISCHARGE_WARN  OutDataTypeStr=boolean
  Energy_Trip_OR : Logic  Operator=OR  IconShape=distinctive
  IL_Meas_Sample : ZeroOrderHold  SampleTime=EP_TS
  IL_Squared : Product
  Ibat_Meas_Sample : ZeroOrderHold  SampleTime=EP_TS
  Ibat_True_Sample : ZeroOrderHold  SampleTime=EP_TS
  Ibus_Source_Sample : ZeroOrderHold  SampleTime=EP_TS
  Iload_Meas_Sample : ZeroOrderHold  SampleTime=EP_TS
  Inductor_Energy : Gain  Gain=0.5*FD_L_MAIN
  Negate_Pbat : Gain  Gain=-1
  Negate_SOC : Gain  Gain=-1
  Pbat_Direction : Gain  Gain=EP_PBAT_SIGN
  Pbat_Meas_Filter : DiscreteTransferFcn  Numerator=1-EP_POWER_ALPHA  Denominator=[1 -EP_POWER_ALPHA]  SampleTime=EP_TS
  Pbat_Measured_Product : Product  Inputs=**
  Pbat_True_Filter : DiscreteTransferFcn  LoadFcn=dspblkCoreblockFVToolHelper(gcbh,'load');  Numerator=1-EP_POWER_ALPHA  Denominator=[1 -EP_POWER_ALPHA]  SampleTime=EP_TS
      settings: CopyFcn=dspblkCoreblockFVToolHelper(gcbh,'copy');  DeleteFcn=dspblkCoreblockFVToolHelper(gcbh,'close');  ModelCloseFcn=dspblkCoreblockFVToolHelper(gcbh,'close');  PreSaveFcn=dspblkCoreblockFVToolHelper(gcbh,'presave');  PostSaveFcn=dspblkCoreblockFVToolHelper(gcbh,'postsave');  CloseFcn=dspblkCoreblockFVToolHelper(gcbh,'close');
  Pbat_True_Product : Product  Inputs=**
  Pload_Direction : Gain  Gain=EP_PLOAD_SIGN
  Pload_Measured_Product : Product
  Power_Balance_Residual : Sum  Inputs=+-
  Power_Confirm_Timer : DiscreteIntegrator  gainval=1  ExternalReset=falling  SampleTime=EP_TS  LimitOutput=on  UpperSaturationLimit=EP_POWER_CONFIRM_TIME  LowerSaturationLimit=0  ICPrevOutput=DiscIntNeverNeededParam  ICPrevScaledInput=DiscIntNeverNeededParam
  Power_Exceeded_Double : DataTypeConversion  OutDataTypeStr=double
  Power_Exceeded_OR : Logic  Operator=OR  IconShape=distinctive
  Power_Injected_Sum : Sum  Inputs=+++
  Power_Trip_Confirmed : hdlsllib/Logic and Bit Operations/Compare To Constant  relop=>=  const=EP_POWER_CONFIRM_TIME  OutDataTypeStr=boolean
  Power_Warning_OR : Logic  Operator=OR  IconShape=distinctive
  Psource_Direction : Gain  Gain=EP_PSOURCE_SIGN
  Psource_Measured_Product : Product
  SOC_Above_Range : hdlsllib/Logic and Bit Operations/Compare To Constant  relop=>  const=100  OutDataTypeStr=boolean
  SOC_Below_Range : hdlsllib/Logic and Bit Operations/Compare To Constant  relop=<  const=0  OutDataTypeStr=boolean
  SOC_High_Warning : hdlsllib/Logic and Bit Operations/Compare To Constant  relop=>=  const=EP_SOC_WARN_HIGH  OutDataTypeStr=boolean
  SOC_Invalid_OR : Logic  Operator=OR  IconShape=distinctive
  SOC_Low_Warning : hdlsllib/Logic and Bit Operations/Compare To Constant  relop=<=  const=EP_SOC_WARN_LOW  OutDataTypeStr=boolean
  SOC_Sample : ZeroOrderHold  SampleTime=EP_TS
  SOC_Warning_OR : Logic  Operator=OR  IconShape=distinctive
  Stored_Energy : Sum
  Stored_Energy_Delta : Sum  Inputs=+-
  Stored_Energy_Previous : UnitDelay  InitialCondition=EP_ENERGY_INITIAL  SampleTime=EP_TS
  Stored_Power_Derivative : Gain  Gain=1/EP_TS
  Stored_Power_Filter : DiscreteTransferFcn  Numerator=1-EP_POWER_BALANCE_ALPHA  Denominator=[1 -EP_POWER_BALANCE_ALPHA]  SampleTime=EP_TS
  Vbat_Meas_Sample : ZeroOrderHold  SampleTime=EP_TS
  Vbat_True_Sample : ZeroOrderHold  SampleTime=EP_TS
  Vbus_Meas_Sample : ZeroOrderHold  SampleTime=EP_TS
  Vbus_Squared : Product
  charge_allowed : Outport
  discharge_allowed : Outport  Port=2
  soc_warning : Outport  Port=3
  power_warning : Outport  Port=4
  energy_trip_request : Outport  Port=5
  Pbat_meas : Outport  Port=6
  Pbat_true : Outport  Port=7
  Pcharge : Outport  Port=8
  Pdischarge : Outport  Port=9
  Psource_meas : Outport  Port=10
  Pload_meas : Outport  Port=11
  Pstored_meas : Outport  Port=12
  PowerBalanceResidual : Outport  Port=13
  wires:
  Energy_Trip_OR/1 -> energy_trip_request/1
  SOC_Invalid_OR/1 -> Energy_Trip_OR/2
  Power_Trip_Confirmed/1 -> Energy_Trip_OR/1
  Power_Confirm_Timer/1 -> Power_Trip_Confirmed/1
  Power_Exceeded_Double/1 -> Power_Confirm_Timer/1, Power_Confirm_Timer/2
  Power_Exceeded_OR/1 -> Power_Exceeded_Double/1
  Discharge_Power_Exceeded/1 -> Power_Exceeded_OR/2
  Charge_Power_Exceeded/1 -> Power_Exceeded_OR/1
  Power_Warning_OR/1 -> power_warning/1
  Discharge_Power_Warning/1 -> Power_Warning_OR/2
  Charge_Power_Warning/1 -> Power_Warning_OR/1
  Discharge_Power_Positive/1 -> Discharge_Power_Exceeded/1, Pdischarge/1, Discharge_Power_Warning/1
  Charge_Power_Positive/1 -> Pcharge/1, Charge_Power_Warning/1, Charge_Power_Exceeded/1
  Negate_Pbat/1 -> Charge_Power_Positive/1
  Pbat_True_Filter/1 -> Pbat_true/1
  Pbat_Meas_Filter/1 -> Discharge_Power_Positive/1, Pbat_meas/1, Pbat_Direction/1, Negate_Pbat/1
  Pbat_True_Product/1 -> Pbat_True_Filter/1
  Pbat_Measured_Product/1 -> Pbat_Meas_Filter/1
  Ibat_True_Sample/1 -> Pbat_True_Product/2
  Vbat_True_Sample/1 -> Pbat_True_Product/1
  Ibat_Meas_Sample/1 -> Pbat_Measured_Product/2
  Vbat_Meas_Sample/1 -> Pbat_Measured_Product/1
  SOC_Below_Range/1 -> SOC_Invalid_OR/2
  SOC_Above_Range/1 -> SOC_Invalid_OR/1
  SOC_Warning_OR/1 -> soc_warning/1
  SOC_Low_Warning/1 -> SOC_Warning_OR/2
  SOC_High_Warning/1 -> SOC_Warning_OR/1
  Discharge_Allowed_Relay/1 -> discharge_allowed/1
  Charge_Allowed_Relay/1 -> charge_allowed/1
  Negate_SOC/1 -> Charge_Allowed_Relay/1
  SOC_Sample/1 -> Discharge_Allowed_Relay/1, SOC_Low_Warning/1, SOC_Above_Range/1, SOC_Below_Range/1, Negate_SOC/1, SOC_High_Warning/1
  Ibat_true/1 -> Ibat_True_Sample/1
  Vbat_true/1 -> Vbat_True_Sample/1
  Ibat_meas/1 -> Ibat_Meas_Sample/1
  Vbat_meas/1 -> Vbat_Meas_Sample/1
  SOC/1 -> SOC_Sample/1
  Ibus_source/1 -> Ibus_Source_Sample/1
  Vbus_meas/1 -> Vbus_Meas_Sample/1
  Iload_meas/1 -> Iload_Meas_Sample/1
  IL_meas/1 -> IL_Meas_Sample/1
  Vbus_Meas_Sample/1 -> Vbus_Squared/2, Psource_Measured_Product/1, Vbus_Squared/1, Pload_Measured_Product/1
  Ibus_Source_Sample/1 -> Psource_Measured_Product/2
  Iload_Meas_Sample/1 -> Pload_Measured_Product/2
  Psource_Measured_Product/1 -> Psource_meas/1, Psource_Direction/1
  Pload_Measured_Product/1 -> Pload_meas/1, Pload_Direction/1
  Vbus_Squared/1 -> Bus_Capacitor_Energy/1
  IL_Meas_Sample/1 -> IL_Squared/2, IL_Squared/1
  IL_Squared/1 -> Inductor_Energy/1
  Bus_Capacitor_Energy/1 -> Stored_Energy/1
  Inductor_Energy/1 -> Stored_Energy/2
  Stored_Energy/1 -> Stored_Energy_Delta/1, Stored_Energy_Previous/1
  Stored_Energy_Previous/1 -> Stored_Energy_Delta/2
  Stored_Energy_Delta/1 -> Stored_Power_Derivative/1
  Stored_Power_Derivative/1 -> Stored_Power_Filter/1
  Psource_Direction/1 -> Power_Injected_Sum/1
  Pbat_Direction/1 -> Power_Injected_Sum/2
  Pload_Direction/1 -> Power_Injected_Sum/3
  Power_Injected_Sum/1 -> Power_Balance_Residual/1
  Stored_Power_Filter/1 -> Pstored_meas/1, Power_Balance_Residual/2
  Power_Balance_Residual/1 -> PowerBalanceResidual/1

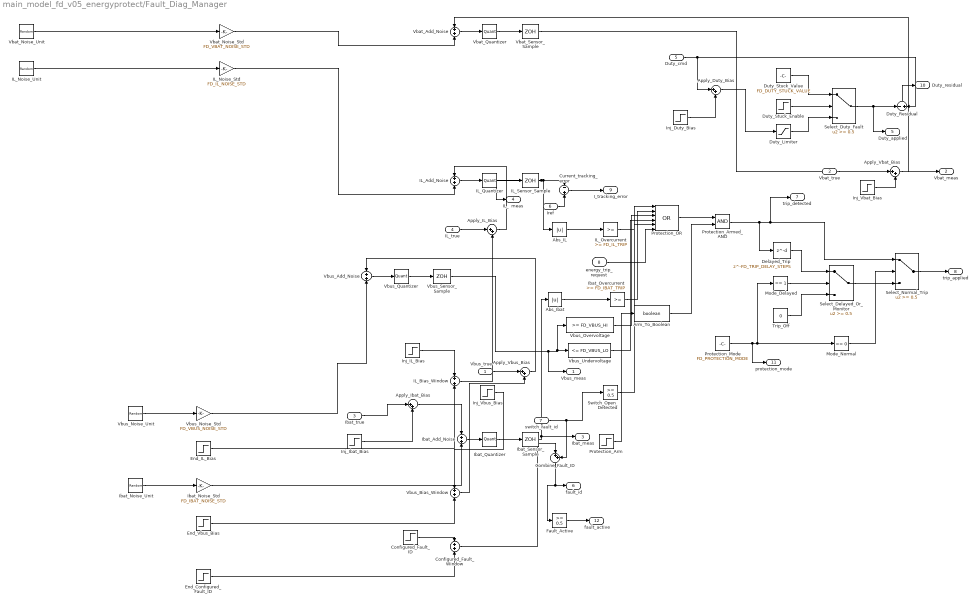
== system main_model_fd_v05_energyprotect/Fault_Diag_Manager ==
  Vbus_true : Inport
  Vbat_true : Inport  Port=2
  Ibat_true : Inport  Port=3
  IL_true : Inport  Port=4
  Duty_cmd : Inport  Port=5
  Iref : Inport  Port=6
  switch_fault_id : Inport  Port=7
  energy_trip_request : Inport  Port=8
  Abs_IL : Abs
  Abs_Ibat : Abs
  Apply_Duty_Bias : Sum  Inputs=|++
  Apply_IL_Bias : Sum  Inputs=|++
  Apply_Ibat_Bias : Sum  Inputs=|++
  Apply_Vbat_Bias : Sum  Inputs=|++
  Apply_Vbus_Bias : Sum  Inputs=|++
  Arm_To_Boolean : DataTypeConversion  OutDataTypeStr=boolean
  Combine_Fault_ID : Sum  Inputs=|++
  Configured_Fault_ID : Step  Time=FD_FAULT_TIME  After=FD_FAULT_ID  SampleTime=FD_TS
  Configured_Fault_Window : Sum
  Current_tracking_error : Sum  Inputs=-+
  Delayed_Trip : Delay  DelayLength=FD_TRIP_DELAY_STEPS  DelayLengthUpperLimit=200000  InitialCondition=0  UseCircularBuffer=on  SampleTime=FD_TS
  Duty_Limiter : Saturate  UpperLimit=1  LowerLimit=0
  Duty_Residual : Sum  Inputs=-+
  Duty_Stuck_Enable : Step  Time=FD_FAULT_TIME  After=FD_DUTY_STUCK_ENABLE  SampleTime=FD_TS
  Duty_Stuck_Value : Constant  Value=FD_DUTY_STUCK_VALUE
  End_Configured_Fault_ID : Step  Time=FD_FAULT_END_TIME  After=-FD_FAULT_ID  SampleTime=FD_TS
  End_IL_Bias : Step  Time=FD_FAULT_END_TIME  After=-FD_IL_BIAS  SampleTime=FD_TS
  End_Vbus_Bias : Step  Time=FD_FAULT_END_TIME  After=-FD_VBUS_BIAS  SampleTime=FD_TS
  Fault_Active : hdlsllib/Logic and Bit Operations/Compare To Constant  relop=>=  const=0.5  OutDataTypeStr=boolean
  IL_Add_Noise : Sum
  IL_Bias_Window : Sum
  IL_Noise_Std : Gain  Gain=FD_IL_NOISE_STD
  IL_Noise_Unit : RandomNumber  Seed=RandomSeed+14  SampleTime=FD_SENSOR_TS
  IL_Overcurrent : hdlsllib/Logic and Bit Operations/Compare To Constant  relop=>=  const=FD_IL_TRIP  OutDataTypeStr=boolean
  IL_Quantizer : Quantizer  QuantizationInterval=FD_CURRENT_QUANT_STEP
  IL_Sensor_Sample : ZeroOrderHold  SampleTime=FD_SENSOR_TS
  Ibat_Add_Noise : Sum
  Ibat_Noise_Std : Gain  Gain=FD_IBAT_NOISE_STD
  Ibat_Noise_Unit : RandomNumber  Seed=RandomSeed+13  SampleTime=FD_SENSOR_TS
  Ibat_Overcurrent : hdlsllib/Logic and Bit Operations/Compare To Constant  relop=>=  const=FD_IBAT_TRIP  OutDataTypeStr=boolean
  Ibat_Quantizer : Quantizer  QuantizationInterval=FD_CURRENT_QUANT_STEP
  Ibat_Sensor_Sample : ZeroOrderHold  SampleTime=FD_SENSOR_TS
  Inj_Duty_Bias : Step  Time=FD_FAULT_TIME  After=FD_DUTY_BIAS  SampleTime=FD_TS
  Inj_IL_Bias : Step  Time=FD_FAULT_TIME  After=FD_IL_BIAS  SampleTime=FD_TS
  Inj_Ibat_Bias : Step  Time=FD_FAULT_TIME  After=FD_IBAT_BIAS  SampleTime=FD_TS
  Inj_Vbat_Bias : Step  Time=FD_FAULT_TIME  After=FD_VBAT_BIAS  SampleTime=FD_TS
  Inj_Vbus_Bias : Step  Time=FD_FAULT_TIME  After=FD_VBUS_BIAS  SampleTime=FD_TS
  Mode_Delayed : hdlsllib/Logic and Bit Operations/Compare To Constant  relop===  const=1  OutDataTypeStr=boolean
  Mode_Normal : hdlsllib/Logic and Bit Operations/Compare To Constant  relop===  const=0  OutDataTypeStr=boolean
  Protection_Arm : Step  Time=FD_PROTECTION_ARM_TIME  SampleTime=FD_TS
  Protection_Armed_AND : Logic  OutDataTypeStr=boolean
  Protection_Mode : Constant  Value=FD_PROTECTION_MODE
  Protection_OR : Logic  Operator=OR  Inputs=6  OutDataTypeStr=boolean
  Select_Delayed_Or_Monitor : Switch  Threshold=0.5
  Select_Duty_Fault : Switch  Threshold=0.5
  Select_Normal_Trip : Switch  Threshold=0.5
  Switch_Open_Detected : hdlsllib/Logic and Bit Operations/Compare To Constant  relop=>=  const=0.5  OutDataTypeStr=boolean
  Trip_Off : Constant  Value=0  OutDataTypeStr=boolean
  Vbat_Add_Noise : Sum
  Vbat_Noise_Std : Gain  Gain=FD_VBAT_NOISE_STD
  Vbat_Noise_Unit : RandomNumber  Seed=RandomSeed+12  SampleTime=FD_SENSOR_TS
  Vbat_Quantizer : Quantizer  QuantizationInterval=FD_VBAT_QUANT_STEP
  Vbat_Sensor_Sample : ZeroOrderHold  SampleTime=FD_SENSOR_TS
  Vbus_Add_Noise : Sum
  Vbus_Bias_Window : Sum
  Vbus_Noise_Std : Gain  Gain=FD_VBUS_NOISE_STD
  Vbus_Noise_Unit : RandomNumber  Seed=RandomSeed+11  SampleTime=FD_SENSOR_TS
  Vbus_Overvoltage : hdlsllib/Logic and Bit Operations/Compare To Constant  relop=>=  const=FD_VBUS_HI  OutDataTypeStr=boolean
  Vbus_Quantizer : Quantizer  QuantizationInterval=FD_VBUS_QUANT_STEP
  Vbus_Sensor_Sample : ZeroOrderHold  SampleTime=FD_SENSOR_TS
  Vbus_Undervoltage : hdlsllib/Logic and Bit Operations/Compare To Constant  relop=<=  const=FD_VBUS_LO  OutDataTypeStr=boolean
  Vbus_meas : Outport
  Vbat_meas : Outport  Port=2
  Ibat_meas : Outport  Port=3
  IL_  meas : Outport  Port=4
  Duty_applied : Outport  Port=5
  fault_id : Outport  Port=6
  trip_detected : Outport  Port=7
  trip_applied : Outport  Port=8
  I_tracking_error : Outport  Port=9
  Duty_residual : Outport  Port=10
  protection_mode : Outport  Port=11
  fault_active : Outport  Port=12
  wires:
  Duty_Residual/1 -> Duty_residual/1
  Current_tracking_error/1 -> I_tracking_error/1
  Iref/1 -> Current_tracking_error/2
  Fault_Active/1 -> fault_active/1
  Combine_Fault_ID/1 -> fault_id/1, Fault_Active/1
  switch_fault_id/1 -> Combine_Fault_ID/2, Switch_Open_Detected/1
  Select_Duty_Fault/1 -> Duty_applied/1, Duty_Residual/1
  Duty_Limiter/1 -> Select_Duty_Fault/3
  Duty_Stuck_Enable/1 -> Select_Duty_Fault/2
  Duty_Stuck_Value/1 -> Select_Duty_Fault/1
  Apply_Duty_Bias/1 -> Duty_Limiter/1
  Inj_Duty_Bias/1 -> Apply_Duty_Bias/2
  Duty_cmd/1 -> Apply_Duty_Bias/1, Duty_Residual/2
  IL_true/1 -> Apply_IL_Bias/1
  Inj_Ibat_Bias/1 -> Apply_Ibat_Bias/2
  Ibat_true/1 -> Apply_Ibat_Bias/1
  Inj_Vbat_Bias/1 -> Apply_Vbat_Bias/2
  Vbat_true/1 -> Apply_Vbat_Bias/1
  Vbus_true/1 -> Apply_Vbus_Bias/1
  Abs_IL/1 -> IL_Overcurrent/1
  Abs_Ibat/1 -> Ibat_Overcurrent/1
  IL_Overcurrent/1 -> Protection_OR/1
  Ibat_Overcurrent/1 -> Protection_OR/2
  Vbus_Overvoltage/1 -> Protection_OR/3
  Vbus_Undervoltage/1 -> Protection_OR/4
  Switch_Open_Detected/1 -> Protection_OR/5
  Protection_OR/1 -> Protection_Armed_AND/1
  Protection_Armed_AND/1 -> trip_detected/1, Select_Normal_Trip/1, Delayed_Trip/1
  Delayed_Trip/1 -> Select_Delayed_Or_Monitor/1
  Protection_Mode/1 -> Mode_Delayed/1, Mode_Normal/1, protection_mode/1
  Mode_Delayed/1 -> Select_Delayed_Or_Monitor/2
  Trip_Off/1 -> Select_Delayed_Or_Monitor/3
  Mode_Normal/1 -> Select_Normal_Trip/2
  Select_Delayed_Or_Monitor/1 -> Select_Normal_Trip/3
  Select_Normal_Trip/1 -> trip_applied/1
  Protection_Arm/1 -> Arm_To_Boolean/1
  Arm_To_Boolean/1 -> Protection_Armed_AND/2
  energy_trip_request/1 -> Protection_OR/6
  Inj_Vbus_Bias/1 -> Vbus_Bias_Window/1
  End_Vbus_Bias/1 -> Vbus_Bias_Window/2
  Vbus_Bias_Window/1 -> Apply_Vbus_Bias/2
  Inj_IL_Bias/1 -> IL_Bias_Window/1
  End_IL_Bias/1 -> IL_Bias_Window/2
  IL_Bias_Window/1 -> Apply_IL_Bias/2
  Configured_Fault_ID/1 -> Configured_Fault_Window/1
  End_Configured_Fault_ID/1 -> Configured_Fault_Window/2
  Configured_Fault_Window/1 -> Combine_Fault_ID/1
  Apply_Vbus_Bias/1 -> Vbus_Add_Noise/1
  Vbus_Noise_Unit/1 -> Vbus_Noise_Std/1
  Vbus_Noise_Std/1 -> Vbus_Add_Noise/2
  Vbus_Add_Noise/1 -> Vbus_Quantizer/1
  Vbus_Quantizer/1 -> Vbus_Sensor_Sample/1
  Vbus_Sensor_Sample/1 -> Vbus_meas/1, Vbus_Undervoltage/1, Vbus_Overvoltage/1
  Apply_Vbat_Bias/1 -> Vbat_Add_Noise/1
  Vbat_Noise_Unit/1 -> Vbat_Noise_Std/1
  Vbat_Noise_Std/1 -> Vbat_Add_Noise/2
  Vbat_Add_Noise/1 -> Vbat_Quantizer/1
  Vbat_Quantizer/1 -> Vbat_Sensor_Sample/1
  Vbat_Sensor_Sample/1 -> Vbat_meas/1
  Apply_Ibat_Bias/1 -> Ibat_Add_Noise/1
  Ibat_Noise_Unit/1 -> Ibat_Noise_Std/1
  Ibat_Noise_Std/1 -> Ibat_Add_Noise/2
  Ibat_Add_Noise/1 -> Ibat_Quantizer/1
  Ibat_Quantizer/1 -> Ibat_Sensor_Sample/1
  Ibat_Sensor_Sample/1 -> Abs_Ibat/1, Ibat_meas/1
  Apply_IL_Bias/1 -> IL_Add_Noise/1
  IL_Noise_Unit/1 -> IL_Noise_Std/1
  IL_Noise_Std/1 -> IL_Add_Noise/2
  IL_Add_Noise/1 -> IL_Quantizer/1
  IL_Quantizer/1 -> IL_Sensor_Sample/1
  IL_Sensor_Sample/1 -> Current_tracking_error/1, Abs_IL/1, IL_  meas/1

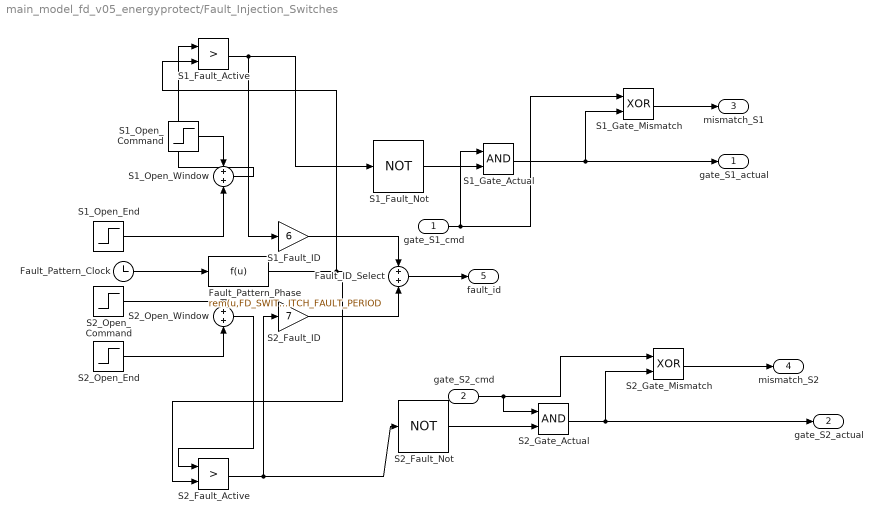
== system main_model_fd_v05_energyprotect/Fault_Injection_Switches ==
  gate_S1_cmd : Inport
  gate_S2_cmd : Inport  Port=2
  Fault_ID_Select : Sum
  Fault_Pattern_Clock : Clock
  Fault_Pattern_Phase : Fcn  Expr=rem(u,FD_SWITCH_FAULT_PERIOD)/FD_SWITCH_FAULT_PERIOD
  S1_Fault_Active : RelationalOperator  Operator=>
  S1_Fault_ID : Gain  Gain=6
  S1_Fault_Not : Logic  Operator=NOT
  S1_Gate_Actual : Logic
  S1_Gate_Mismatch : Logic  Operator=XOR
  S1_Open_Command : Step  Time=FD_FAULT_TIME  After=FD_S1_OPEN  SampleTime=FD_TS
  S1_Open_End : Step  Time=FD_FAULT_END_TIME  After=-FD_S1_OPEN  SampleTime=FD_TS
  S1_Open_Window : Sum
  S2_Fault_Active : RelationalOperator  Operator=>
  S2_Fault_ID : Gain  Gain=7
  S2_Fault_Not : Logic  Operator=NOT
  S2_Gate_Actual : Logic
  S2_Gate_Mismatch : Logic  Operator=XOR
  S2_Open_Command : Step  Time=FD_FAULT_TIME  After=FD_S2_OPEN  SampleTime=FD_TS
  S2_Open_End : Step  Time=FD_FAULT_END_TIME  After=-FD_S2_OPEN  SampleTime=FD_TS
  S2_Open_Window : Sum
  gate_S1_actual : Outport
  gate_S2_actual : Outport  Port=2
  mismatch_S1 : Outport  Port=3
  mismatch_S2 : Outport  Port=4
  fault_id : Outport  Port=5
  wires:
  gate_S1_cmd/1 -> S1_Gate_Actual/1, S1_Gate_Mismatch/1
  S1_Fault_Not/1 -> S1_Gate_Actual/2
  S1_Gate_Actual/1 -> S1_Gate_Mismatch/2, gate_S1_actual/1
  S1_Gate_Mismatch/1 -> mismatch_S1/1
  gate_S2_cmd/1 -> S2_Gate_Actual/1, S2_Gate_Mismatch/1
  S2_Fault_Not/1 -> S2_Gate_Actual/2
  S2_Gate_Actual/1 -> S2_Gate_Mismatch/2, gate_S2_actual/1
  S2_Gate_Mismatch/1 -> mismatch_S2/1
  S1_Fault_ID/1 -> Fault_ID_Select/1
  S2_Fault_ID/1 -> Fault_ID_Select/2
  Fault_ID_Select/1 -> fault_id/1
  S1_Open_End/1 -> S1_Open_Window/2
  S2_Open_End/1 -> S2_Open_Window/2
  S1_Open_Command/1 -> S1_Open_Window/1
  S1_Fault_Active/1 -> S1_Fault_ID/1, S1_Fault_Not/1
  S2_Fault_Active/1 -> S2_Fault_ID/1, S2_Fault_Not/1
  S1_Open_Window/1 -> S1_Fault_Active/1
  S2_Open_Window/1 -> S2_Fault_Active/1
  S2_Open_Command/1 -> S2_Open_Window/1
  Fault_Pattern_Clock/1 -> Fault_Pattern_Phase/1
  Fault_Pattern_Phase/1 -> S2_Fault_Active/2, S1_Fault_Active/2

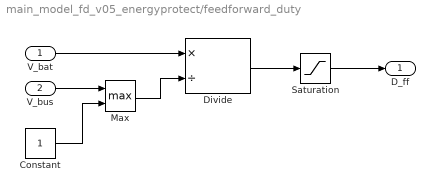
== system main_model_fd_v05_energyprotect/feedforward_duty ==
  V_bat : Inport
  V_bus : Inport  Port=2
  Constant : Constant
  Divide : Product  Inputs=*/
  Max : MinMax  Function=max  Inputs=2
  Saturation : Saturate  UpperLimit=1  LowerLimit=0
  D_ff : Outport
  wires:
  V_bat/1 -> Divide/1
  Divide/1 -> Saturation/1
  Saturation/1 -> D_ff/1
  Max/1 -> Divide/2
  V_bus/1 -> Max/1
  Constant/1 -> Max/2
